simulink model "PowerWindowSystem"  (R2024b)
settings: Solver=VariableStepAuto  StartTime=0.0  StopTime=20  RelTol=1e-3  AbsTol=1e-3  EnableMultiTasking=on
libraries: fl_lib x26, sdl_lib x10, nesl_utility x5
CloseFcn:
  | try,close(h1_PowerWindowSystem),end
  | clear h1_PowerWindowSystem
  | 
  | 
  | clear simlog_PowerWindowSystem
Description:
  | Power Window System
settings Model: Creator=The MathWorks, Inc.  LastModifiedBy=linus
settings SolverCC: AutoScaleAbsTol=off  MaxConsecutiveMinStep=5  AlgebraicLoopSolver=TrustRegion  MaxZcPerStep=1
settings DataIOCC: LimitDataPoints=on  MaxDataPoints=10000  SaveFormat=Array  ReturnWorkspaceOutputs=off  SignalLoggingName=logsout_PowerWindowSystem
settings OptimizationCC: ExpressionDepthLimit=2147483647  EfficientMapNaN2IntZero=off  LifeSpan=inf
settings DebuggingCC: UnconnectedInputMsg=warning  UnconnectedOutputMsg=warning  UnconnectedLineMsg=warning  StateNameClashWarn=warning  PregeneratedLibrarySubsystemCodeDiagnostic=none  SFUnexpectedBacktrackingDiag=warning  SFNoUnconditionalDefaultTransitionDiag=warning  SFExecutionAtInitializationDiag=none  ArithmeticOperatorsInVariantConditions=warning
settings HardwareCC: ProdBitPerPointer=32  ProdBitPerSizeT=32  ProdBitPerPtrDiffT=32  ProdLargestAtomicFloat=None  ProdIntDivRoundTo=Undefined  ProdEndianess=Unspecified  ProdWordSize=32  ProdHWDeviceType=32-bit Generic
settings ModelReferenceCC: EnableRefExpFcnMdlSchedulingChecks=on  PropagateSignalLabelsOutOfModel=off
settings SFSimCC: SimUseLocalCustomCode=off  CustomCodeUndefinedFunction=UseInterfaceOnly
settings RTWCC: RTWUseLocalCustomCode=off  GPUComputeCapability=3.5  DLArmComputeVersion=19.05
settings CodeAppCC: StateflowObjectComments=on
settings GRTTargetCC: TargetLangStandard=C89/C90 (ANSI)  CombineOutputUpdateFcns=off  GRTInterface=on
settings ConfigComp: CovMetricSettings=dw  CovSaveCumulativeToWorkspaceVar=on  CovSaveSingleToWorkspaceVar=on  CovExternalEMLEnable=off
settings SimscapeCC: SimscapeLogType=all  SimscapeLogSimulationStatistics=on  SimscapeLogName=simlog_PowerWindowSystem  SimscapeLogDataHistory=20000

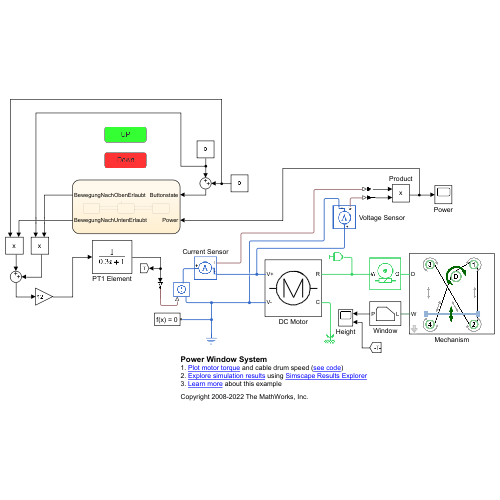
[thumbnail: Simulink's stored preview of the top-level diagram]
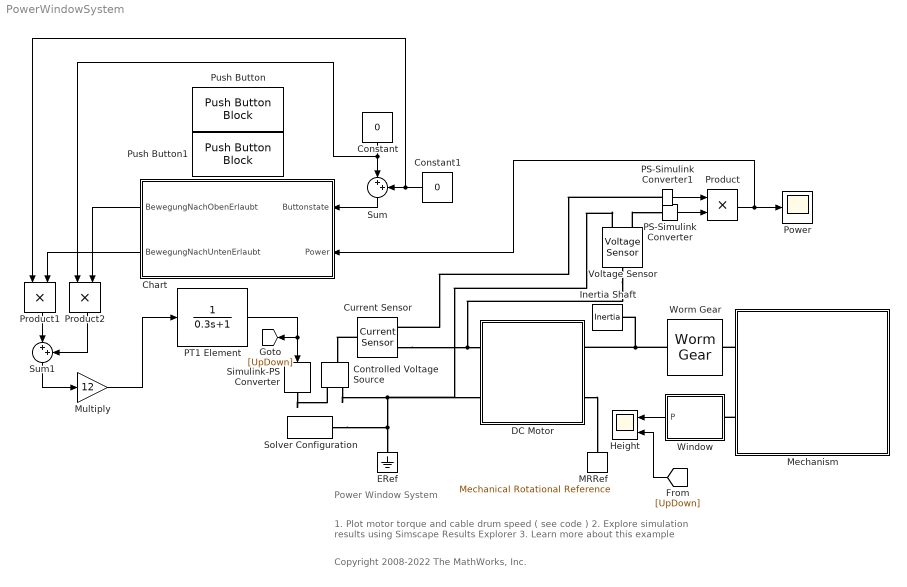
== system PowerWindowSystem ==
  note: Copyright 2008-2022 The MathWorks, Inc.
  note: Power Window System
  note: 1. Plot motor torque and cable drum speed ( see code )
      | 2. Explore simulation results using Simscape Results Explorer
      | 3. Learn more about this example
  Chart : Stateflow chart  TreatAsAtomicUnit=on
      settings: PortSchema="{\"entries\":[{\"content\":{\"sides\":[{\"content\":{\"connectorIds\":[\"In2\",\"In1\"]},\"type\":\"ConnectorPlacement.EquallySpacedRectSide\",\"uuid\":\"8bc5505b-9316-475f-ad7f-30c7afcbaf38\"},{\"content\":{\"connectorIds\":[\"Out1\",\"Out2\"],\"side\":\"RIGHT\"},\"type\":\"ConnectorPlacement.EquallySpacedRectSide\",\"uuid\":\"548d1c51-bdfb-47bd-abc9-5f518f35e423\"},{\"content\":{\"side\":\"TOP\"},\"type\":\"ConnectorPlacement.EquallySpacedRectSide\",\"uuid\":\"81f098c8-4566-4ae4-b1ae-e67fa706afd8\"}]},\"type\":\"ConnectorPlacement.EquallySpacedConnector\",\"uuid\":\"ae74842b-5900-4315-b481-75b4a04e7659\"}],\"packageUris\":[\"http://schema.mathworks.com/mf0/Connector/R2020b\"],\"version\":\"1.0\"}"
  Constant : Constant  Value=0
  Constant1 : Constant  Value=0
  Controlled Voltage Source : fl_lib/Electrical/Electrical Sources/Controlled Voltage Source
  Current Sensor : fl_lib/Electrical/Electrical Sensors/Current Sensor
  DC Motor : Subsystem  Tag=PublishSubsystem
      mask Display:
      | % Circle
      | plot(sin(0:0.1:2.2*pi)*0.9,cos(0:0.1:2.2*pi)*0.9);
      | 
      | % In/out
      | plot([-1.3 -0.9],[0 0]);
      | plot([1.3 0.9],[0 0]);
      | 
      | % 'M'
      | plot([0.5 0.5],[-0.5 0.5]);
      | plot([-0.5 -0.5],[-0.5 0.5]);
      | plot([0.5 0],[0.5 -0.5]);
      | plot([-0.5 0],[0.5 -0.5]);
      | 
      | % Plot points to set plot range
      | color('white');plot(1.5,1.5);plot(-1.5,-1.5)
      | color('black');
  ERef : fl_lib/Electrical/Electrical Elements/Electrical Reference
  Height : Scope  NumInputPorts=2
  Inertia Shaft : fl_lib/Mechanical/Rotational Elements/Inertia  inertia=0.01 kg*m^2  num_ports=foundation.enum.numPorts2.one  w_specify=on  w_priority=High  w=0 rad/s  w_nominal_specify=off  w_nominal_value=1  w_nominal_unit=rad/s  t_specify=off  t_priority=High  t=0 N*m  t_nominal_specify=off  t_nominal_value=1  t_nominal_unit=N*m
  MRRef : fl_lib/Mechanical/Rotational Elements/Mechanical Rotational Reference
  Mechanism : Subsystem  Tag=PublishSubsystem  mask(Power Window Cable Mechanism){pulley_rad=0.015, pulley_bearing_f=0.001, pulley_inertia=0.01, pulley_mus=0.5, pulley_vth=0.001, cable_massperlen=0.6, cable_k=5000, cable_b=500, cable_init_x=0.01, cable_guideway_f=10, drum_rad=0.030, drum_bearing_f=0.001*0.5}
      mask prompts: pulley_rad "Radius (m)"; pulley_bearing_f "Bearing Friction (N*m/(rad/s))"; pulley_inertia "Inertia (kg*m^2)"; pulley_mus "Static Friction with Belt"; pulley_vth "Friction Velocity Thresh. (m/s)"; cable_massperlen "Mass Per Length (kg/m)"; cable_k "Cable Stiffness (N/m)"; cable_b "Cable Damping (N/(m/s))"; cable_init_x "Cable Initial Deformation (m)"; cable_guideway_f "Guideway Friction (N/(m/s))"; drum_rad "Radius (m)"; drum_bearing_f "Bearing Friction (N*m/(rad/s))"
      mask help: Represents cable mechanism for raising and lowering a window. A cable is routed around four pulleys such that both ends of a lift plate can be raised and lowered. The mechanism is actuated by rotating the shaft of a rope drum.
      mask DialogControl Container28 Prompt: Pulley
      mask DialogControl Container25 Prompt: Cable
      mask DialogControl Container25_copy Prompt: Drum
      mask Display: image('PowerWindowSystemMechanismSchematic.jpg','center');
  Multiply : Gain  Gain=12
  PS-Simulink Converter : nesl_utility/PS-Simulink Converter  PhysicalDomain=network_engine_domain  SubClassName=ps_output  LeftPortType=input  RightPortType=output  PseudoPeriodic=off  Frequencies=[]  VectorFormat=inherit  Unit=inherit  AffineConversion=off
  PS-Simulink Converter1 : nesl_utility/PS-Simulink Converter  PhysicalDomain=network_engine_domain  SubClassName=ps_output  LeftPortType=input  RightPortType=output  PseudoPeriodic=off  Frequencies=[]  VectorFormat=inherit  Unit=inherit  AffineConversion=off
  PT1 Element : TransferFcn  Denominator=[0.3 1]
  Power : Scope
  Product : Product
  Product1 : Product
  Product2 : Product
  Push Button : PushButtonBlock  ButtonText=UP  OnValue=-1  OffValue=0.000000
  Push Button1 : PushButtonBlock  ButtonText=Down  OffValue=0.000000
  Simulink-PS Converter : nesl_utility/Simulink-PS Converter  PhysicalDomain=network_engine_domain  SubClassName=ps_input  LeftPortType=input  RightPortType=output  PseudoPeriodic=off  Frequencies=[]  NoiseDistribution=none  NoiseParameters=[]  Unit=V  AffineConversion=off  FilteringAndDerivatives=filter  SimscapeFilterOrder=1  InputFilterTimeConstant=0.1  UdotUserProvided=1
  Solver Configuration : nesl_utility/Solver Configuration  PhysicalDomain=network_engine_domain  SubClassName=solver  LeftPortType=input  RightPortType=generic  Tones=[]  Harmonics=[]  SimulateNoise=off  Profile=off  UseLocalSampling=off  EnableSwitchedLinearOptims=on  FrequencyDomain=off  UseCCode=off  RelTol=0.001  AbsTol=1e-06  MinStep=1e-09  ToWorkspace=off  RevertToSquareIcSolve=off  NumHomotopyIterations=100  PhasorMode=off  PhasorModeNumHarmonics=1  ConsistencySolver=NEWTON_XTOL_AFTER_FTOL  IndexReductionMethod=DerivativeReplacement  DoDC=off  ResidualTolerance=1e-9  ConsistencyTolSource=GLOBAL  ConsistencyAbsTol=0.001  ConsistencyRelTol=0.001  ConsistencyTolFactor=0.001  UseLocalSolver=off  LocalSolverChoice=NE_PARTITIONING_ADVANCER  ResolveIndetEquations=on  FunctionEvalNumThread=1  LocalSolverSampleTime=.001  DoFixedCost=off  MaxNonlinIter=6  MaxModeIter=2  ComputeImpulses=off  ImpulseIterations=2  LinearAlgebra=auto  LinearAlgebraNumThread=0  EquationFormulation=NE_TIME_EF  DelaysMemoryBudget=1024  AutomaticFiltering=on  FilteringTimeConstant=0.001  PartitionStorageMethod=EXHAUSTIVE  PartitionMemoryBudget=1024  PartitionMethod=ROBUST  MultibodyUseLocalSolver=off  MultibodyLocalSolverChoice=ODE1  MultibodyLocalSolverSampleTime=0.001
  Sum : Sum  Inputs=|++
  Sum1 : Sum  Inputs=|++
  Voltage Sensor : fl_lib/Electrical/Electrical Sensors/Voltage Sensor
  Window : Subsystem  Tag=PublishSubsystem
      mask Display:
      | patch([-1 -1 1 1 -1]*10,[-1 1 1 -1 -1]*8,[1 1 1]);
      | 
      | plot([1 -1]*6,[-1 -1]*5)
      | plot([1 1]*6,[-1 0.6]*5);
      | plot([1 0.8]*6,[0.6 0.9]*5);
      | plot([0.8 -0.1]*6,[0.9 0.9]*5);
      | plot([-0.1 -1]*6,[0.9 0]*5);
      | plot([-1 -1]*6,[0 -1]*5);
  Worm Gear : sdl_lib/Gears/Worm Gear  ratio=50  thread_type=1  friction_model=2  friction_parameterization=1  pr_ang=17.5 deg  lead_ang=3 deg  fr_coeff=0.2  eff_wg=0.74  eff_gw=0.65  temperature_TLU=[ 280 300 320 ] K  efficiency_wg_TLU=[ 0.75 0.7 0.65 ]  efficiency_gw_TLU=[ 0.5 0.45 0.4 ]  pwr_thr=0.001 W  mu_visc=[ 0.001 0.001 ] N*m/(rad/s)  thermal_mass=50 J/K  temperature_specify=off  temperature_priority=High  temperature=300 K  temperature_nominal_specify=off  temperature_nominal_value=1  temperature_nominal_unit=K
      settings: InternalSimscapePortConfiguration="{\"Bottom\":[],\"Left\":[{\"id\":\"W\",\"label\":\"W\",\"type\":\"foundation.mechanical.rotational.rotational\"}],\"Right\":[{\"id\":\"G\",\"label\":\"G\",\"type\":\"foundation.mechanical.rotational.rotational\"}],\"Top\":[]}"
  wires:
  Window/1(P) -> Height/1
  [UpDown] -> Height/2
  PS-Simulink Converter1/1 -> Product/1
  PS-Simulink Converter/1 -> Product/2
  Product/1 -> Chart/1(Power), Power/1
  Sum/1 -> Chart/2(Buttonstate)
  Sum1/1 -> Multiply/1
  Constant/1 -> Sum/1, Product2/1
  Constant1/1 -> Product1/1, Sum/2
  Chart/1(BewegungNachObenErlaubt) -> Product2/2
  Chart/2(BewegungNachUntenErlaubt) -> Product1/2
  Product1/1 -> Sum1/1
  Product2/1 -> Sum1/2
  Multiply/1 -> PT1 Element/1
  PT1 Element/1 -> Simulink-PS Converter/1, [UpDown]
  connections:
  Worm Gear/LConn1 -- DC Motor/RConn1 -- Inertia Shaft/LConn1
  Mechanism/LConn1 -- Worm Gear/RConn1
  Mechanism/LConn2 -- Window/LConn1
  DC Motor/RConn2 -- MRRef/LConn1
  Simulink-PS Converter/RConn1 -- Controlled Voltage Source/RConn1
  Controlled Voltage Source/RConn2 -- Voltage Sensor/RConn2 -- DC Motor/LConn2 -- ERef/LConn1 -- Solver Configuration/RConn1
  Voltage Sensor/RConn1 -- PS-Simulink Converter/LConn1
  PS-Simulink Converter1/LConn1 -- Current Sensor/RConn1
  Current Sensor/RConn2 -- Voltage Sensor/LConn1 -- DC Motor/LConn1
  Current Sensor/LConn1 -- Controlled Voltage Source/LConn1

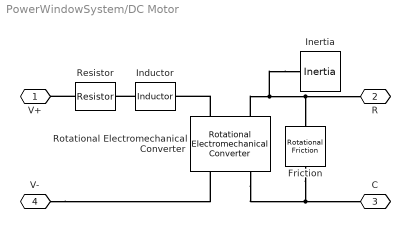
== system PowerWindowSystem/DC Motor ==
  Friction : fl_lib/Mechanical/Rotational Elements/Rotational Friction  brkwy_trq=0.02e-3 N*m  brkwy_vel=0.03347 rad/s  Col_trq=0.02e-3 N*m  visc_coef=.04 N*m/(rad/s)  w_specify=off  w_priority=High  w=0 rad/s  w_nominal_specify=off  w_nominal_value=1  w_nominal_unit=rad/s  t_specify=off  t_priority=High  t=0 N*m  t_nominal_specify=off  t_nominal_value=1  t_nominal_unit=N*m
  Inductor : fl_lib/Electrical/Electrical Elements/Inductor  l=5.5e-5 H  r=0 Ohm  g=1e-09 1/Ohm  i_specify=off  i_priority=High  i=0 A  i_nominal_specify=off  i_nominal_value=1  i_nominal_unit=A  v_specify=off  v_priority=High  v=0 V  v_nominal_specify=off  v_nominal_value=1  v_nominal_unit=V  i_L_specify=off  i_L_priority=High  i_L=0 A  i_L_nominal_specify=off  i_L_nominal_value=1  i_L_nominal_unit=A
  Inertia : fl_lib/Mechanical/Rotational Elements/Inertia  inertia=2.5e-5 g*cm^2  num_ports=foundation.enum.numPorts2.one  w_specify=on  w_priority=None  w=0 rad/s  w_nominal_specify=off  w_nominal_value=1  w_nominal_unit=rad/s  t_specify=off  t_priority=High  t=0 N*m  t_nominal_specify=off  t_nominal_value=1  t_nominal_unit=N*m
  Resistor : fl_lib/Electrical/Electrical Elements/Resistor  Tag=Factory Generic  R=.05 Ohm  i_specify=off  i_priority=High  i=0 A  i_nominal_specify=off  i_nominal_value=1  i_nominal_unit=A  v_specify=off  v_priority=High  v=0 V  v_nominal_specify=off  v_nominal_value=1  v_nominal_unit=V
  Rotational Electromechanical Converter : fl_lib/Electrical/Electrical Elements/Rotational Electromechanical Converter  K=.015 V/rpm  i_specify=off  i_priority=High  i=0 A  i_nominal_specify=off  i_nominal_value=1  i_nominal_unit=A  v_specify=off  v_priority=High  v=0 V  v_nominal_specify=off  v_nominal_value=1  v_nominal_unit=V  t_specify=off  t_priority=High  t=0 N*m  t_nominal_specify=off  t_nominal_value=1  t_nominal_unit=N*m  w_specify=off  w_priority=High  w=0 rad/s  w_nominal_specify=off  w_nominal_value=1  w_nominal_unit=rad/s
  V+ : PMIOPort  Side=Left
  R : PMIOPort  Port=2  Side=Right
  C : PMIOPort  Port=3  Side=Right
  V- : PMIOPort  Port=4  Side=Left
  connections:
  Rotational Electromechanical Converter/RConn2 -- C/RConn1 -- Friction/RConn1
  Inertia/LConn1 -- R/RConn1 -- Friction/LConn1 -- Rotational Electromechanical Converter/LConn2
  Inductor/LConn1 -- Resistor/RConn1
  Resistor/LConn1 -- V+/RConn1
  V-/RConn1 -- Rotational Electromechanical Converter/RConn1
  Rotational Electromechanical Converter/LConn1 -- Inductor/RConn1

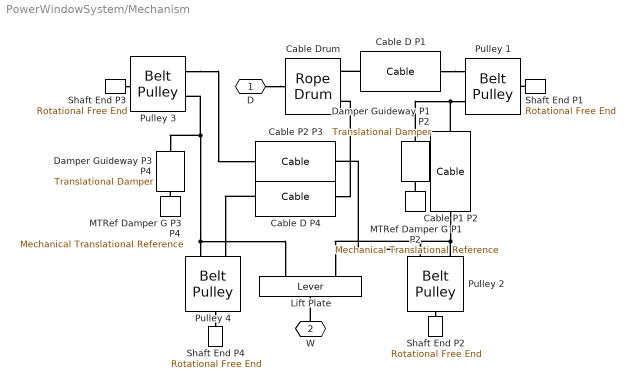
== system PowerWindowSystem/Mechanism ==
  Cable D P1 : sdl_lib/Couplings & Drives/Cable  model_variable_rest_length=false  minimum_rest_length=0.01 m  stretch_parameterization=sdl.enum.CableStretch.Constant  stiffness=cable_k N/m  rigidity=1000 N  damping=cable_b N/(m/s)  stretch_vector=[.1, .2, .5, 1] m  stiffness_vector=[500, 520, 540, 540] N/m  damping_vector=[50, 60, 80, 80] N*s/m  rest_length_vector=[.25, .5, 1] m  stretch_per_rest_length_vector=[.01, .02, .1, .25]  stiffness_table=[500, 600, 600, 500; 250, 300, 300, 250; 125, 150, 150, 125] N/m  damping_table=[50, 60, 60, 50; 50, 60, 60, 50; 50, 60, 60, 50] N*s/m  model_slack=false  slack_model=sdl.enum.SlackBoundary.smooth  transition=0.1 mm  model_mass=simscape.enum.onoff.off  mass=1 kg  linear_density=0.2 kg/m  model_gravity=false  gravity=9.81 m/s^2  theta=0 deg  check_tension=simscape.enum.onoff.on  breakable=sdl.enum.max_tension.off  f_max=1e5 N  s_specify=on  s_priority=High  s=cable_init_x m  s_nominal_specify=off  s_nominal_value=1  s_nominal_unit=m  v_specify=off  v_priority=None  v=0 m/s  v_nominal_specify=off  v_nominal_value=1  v_nominal_unit=m/s  f_specify=off  f_priority=None  f=0 N  f_nominal_specify=off  f_nominal_value=1  f_nominal_unit=N  f_mass_B_specify=off  f_mass_B_priority=None  f_mass_B=0 N  f_mass_B_nominal_specify=off  f_mass_B_nominal_value=1  f_mass_B_nominal_unit=N  f_mass_F_specify=off  f_mass_F_priority=None  f_mass_F=0 N  f_mass_F_nominal_specify=off  f_mass_F_nominal_value=1  f_mass_F_nominal_unit=N
      settings: InternalSimscapePortConfiguration="{\"Bottom\":[],\"Left\":[{\"id\":\"B\",\"label\":\"B\",\"type\":\"foundation.mechanical.translational.translational\"}],\"Right\":[{\"id\":\"F\",\"label\":\"F\",\"type\":\"foundation.mechanical.translational.translational\"}],\"Top\":[]}"
  Cable D P4 : sdl_lib/Couplings & Drives/Cable  model_variable_rest_length=false  minimum_rest_length=0.01 m  stretch_parameterization=sdl.enum.CableStretch.Constant  stiffness=cable_k N/m  rigidity=1000 N  damping=cable_b N/(m/s)  stretch_vector=[.1, .2, .5, 1] m  stiffness_vector=[500, 520, 540, 540] N/m  damping_vector=[50, 60, 80, 80] N*s/m  rest_length_vector=[.25, .5, 1] m  stretch_per_rest_length_vector=[.01, .02, .1, .25]  stiffness_table=[500, 600, 600, 500; 250, 300, 300, 250; 125, 150, 150, 125] N/m  damping_table=[50, 60, 60, 50; 50, 60, 60, 50; 50, 60, 60, 50] N*s/m  model_slack=false  slack_model=sdl.enum.SlackBoundary.smooth  transition=0.1 mm  model_mass=simscape.enum.onoff.off  mass=1 kg  linear_density=0.2 kg/m  model_gravity=false  gravity=9.81 m/s^2  theta=0 deg  check_tension=simscape.enum.onoff.on  breakable=sdl.enum.max_tension.off  f_max=1e5 N  s_specify=on  s_priority=High  s=cable_init_x m  s_nominal_specify=off  s_nominal_value=1  s_nominal_unit=m  v_specify=off  v_priority=None  v=0 m/s  v_nominal_specify=off  v_nominal_value=1  v_nominal_unit=m/s  f_specify=off  f_priority=None  f=0 N  f_nominal_specify=off  f_nominal_value=1  f_nominal_unit=N  f_mass_B_specify=off  f_mass_B_priority=None  f_mass_B=0 N  f_mass_B_nominal_specify=off  f_mass_B_nominal_value=1  f_mass_B_nominal_unit=N  f_mass_F_specify=off  f_mass_F_priority=None  f_mass_F=0 N  f_mass_F_nominal_specify=off  f_mass_F_nominal_value=1  f_mass_F_nominal_unit=N
      settings: InternalSimscapePortConfiguration="{\"Bottom\":[],\"Left\":[{\"id\":\"B\",\"label\":\"B\",\"type\":\"foundation.mechanical.translational.translational\"}],\"Right\":[{\"id\":\"F\",\"label\":\"F\",\"type\":\"foundation.mechanical.translational.translational\"}],\"Top\":[]}"
  Cable Drum : sdl_lib/Couplings & Drives/Rope Drum  r_drum=drum_rad m  windup=sdl.enum.belt_direction.same  check_tension=sdl.enum.tension_check.off  b_drum=drum_bearing_f N*m/(rad/s)  model_inertia=sdl.enum.model_inertia.off  inertia=0.01 kg*m^2  initial_velocity=0 rad/s
      settings: InternalSimscapePortConfiguration="{\"Bottom\":[],\"Left\":[{\"id\":\"S\",\"label\":\"S\",\"type\":\"foundation.mechanical.rotational.rotational\"}],\"Right\":[{\"id\":\"A\",\"label\":\"A\",\"type\":\"foundation.mechanical.translational.translational\"},{\"id\":\"B\",\"label\":\"B\",\"type\":\"foundation.mechanical.translational.translational\"}],\"Top\":[]}"
  Cable P1 P2 : sdl_lib/Couplings & Drives/Cable  model_variable_rest_length=false  minimum_rest_length=0.01 m  stretch_parameterization=sdl.enum.CableStretch.Constant  stiffness=cable_k N/m  rigidity=1000 N  damping=cable_b N/(m/s)  stretch_vector=[.1, .2, .5, 1] m  stiffness_vector=[500, 520, 540, 540] N/m  damping_vector=[50, 60, 80, 80] N*s/m  rest_length_vector=[.25, .5, 1] m  stretch_per_rest_length_vector=[.01, .02, .1, .25]  stiffness_table=[500, 600, 600, 500; 250, 300, 300, 250; 125, 150, 150, 125] N/m  damping_table=[50, 60, 60, 50; 50, 60, 60, 50; 50, 60, 60, 50] N*s/m  model_slack=false  slack_model=sdl.enum.SlackBoundary.smooth  transition=0.1 mm  model_mass=simscape.enum.onoff.off  mass=1 kg  linear_density=0.2 kg/m  model_gravity=false  gravity=9.81 m/s^2  theta=0 deg  check_tension=simscape.enum.onoff.on  breakable=sdl.enum.max_tension.off  f_max=1e5 N  s_specify=on  s_priority=High  s=cable_init_x m  s_nominal_specify=off  s_nominal_value=1  s_nominal_unit=m  v_specify=off  v_priority=None  v=0 m/s  v_nominal_specify=off  v_nominal_value=1  v_nominal_unit=m/s  f_specify=off  f_priority=None  f=0 N  f_nominal_specify=off  f_nominal_value=1  f_nominal_unit=N  f_mass_B_specify=off  f_mass_B_priority=None  f_mass_B=0 N  f_mass_B_nominal_specify=off  f_mass_B_nominal_value=1  f_mass_B_nominal_unit=N  f_mass_F_specify=off  f_mass_F_priority=None  f_mass_F=0 N  f_mass_F_nominal_specify=off  f_mass_F_nominal_value=1  f_mass_F_nominal_unit=N
      settings: InternalSimscapePortConfiguration="{\"Bottom\":[],\"Left\":[{\"id\":\"B\",\"label\":\"B\",\"type\":\"foundation.mechanical.translational.translational\"}],\"Right\":[{\"id\":\"F\",\"label\":\"F\",\"type\":\"foundation.mechanical.translational.translational\"}],\"Top\":[]}"
  Cable P2 P3 : sdl_lib/Couplings & Drives/Cable  model_variable_rest_length=false  minimum_rest_length=0.01 m  stretch_parameterization=sdl.enum.CableStretch.Constant  stiffness=cable_k N/m  rigidity=1000 N  damping=cable_b N/(m/s)  stretch_vector=[.1, .2, .5, 1] m  stiffness_vector=[500, 520, 540, 540] N/m  damping_vector=[50, 60, 80, 80] N*s/m  rest_length_vector=[.25, .5, 1] m  stretch_per_rest_length_vector=[.01, .02, .1, .25]  stiffness_table=[500, 600, 600, 500; 250, 300, 300, 250; 125, 150, 150, 125] N/m  damping_table=[50, 60, 60, 50; 50, 60, 60, 50; 50, 60, 60, 50] N*s/m  model_slack=false  slack_model=sdl.enum.SlackBoundary.smooth  transition=0.1 mm  model_mass=simscape.enum.onoff.off  mass=1 kg  linear_density=0.2 kg/m  model_gravity=false  gravity=9.81 m/s^2  theta=0 deg  check_tension=false  breakable=sdl.enum.max_tension.off  f_max=1e5 N  s_specify=on  s_priority=High  s=cable_init_x m  s_nominal_specify=off  s_nominal_value=1  s_nominal_unit=m  v_specify=off  v_priority=None  v=0 m/s  v_nominal_specify=off  v_nominal_value=1  v_nominal_unit=m/s  f_specify=off  f_priority=None  f=0 N  f_nominal_specify=off  f_nominal_value=1  f_nominal_unit=N  f_mass_B_specify=off  f_mass_B_priority=None  f_mass_B=0 N  f_mass_B_nominal_specify=off  f_mass_B_nominal_value=1  f_mass_B_nominal_unit=N  f_mass_F_specify=off  f_mass_F_priority=None  f_mass_F=0 N  f_mass_F_nominal_specify=off  f_mass_F_nominal_value=1  f_mass_F_nominal_unit=N
      settings: InternalSimscapePortConfiguration="{\"Bottom\":[],\"Left\":[{\"id\":\"B\",\"label\":\"B\",\"type\":\"foundation.mechanical.translational.translational\"}],\"Right\":[{\"id\":\"F\",\"label\":\"F\",\"type\":\"foundation.mechanical.translational.translational\"}],\"Top\":[]}"
  Damper Guideway P1 P2 : fl_lib/Mechanical/Translational Elements/Translational Damper  D=cable_guideway_f N/(m/s)  v_specify=off  v_priority=High  v=0 m/s  v_nominal_specify=off  v_nominal_value=1  v_nominal_unit=m/s  f_specify=off  f_priority=High  f=0 N  f_nominal_specify=off  f_nominal_value=1  f_nominal_unit=N
  Damper Guideway P3 P4 : fl_lib/Mechanical/Translational Elements/Translational Damper  D=cable_guideway_f N/(m/s)  v_specify=off  v_priority=High  v=0 m/s  v_nominal_specify=off  v_nominal_value=1  v_nominal_unit=m/s  f_specify=off  f_priority=High  f=0 N  f_nominal_specify=off  f_nominal_value=1  f_nominal_unit=N
  Lift Plate : fl_lib/Mechanical/Mechanisms/Lever  arm_AC=0.25 m  arm_BC=0.25 m  f_A_specify=off  f_A_priority=High  f_A=0 N  f_A_nominal_specify=off  f_A_nominal_value=1  f_A_nominal_unit=N  f_B_specify=off  f_B_priority=High  f_B=0 N  f_B_nominal_specify=off  f_B_nominal_value=1  f_B_nominal_unit=N  f_C_specify=off  f_C_priority=High  f_C=0 N  f_C_nominal_specify=off  f_C_nominal_value=1  f_C_nominal_unit=N
      settings: InternalSimscapePortConfiguration="{\"Bottom\":[],\"Left\":[{\"id\":\"A\",\"label\":\"A\",\"type\":\"foundation.mechanical.translational.translational\"},{\"id\":\"B\",\"label\":\"B\",\"type\":\"foundation.mechanical.translational.translational\"}],\"Right\":[{\"id\":\"C\",\"label\":\"C\",\"type\":\"foundation.mechanical.translational.translational\"}],\"Top\":[]}"
  MTRef Damper G P1 P2 : fl_lib/Mechanical/Translational Elements/Mechanical Translational Reference
  MTRef Damper G P3 P4 : fl_lib/Mechanical/Translational Elements/Mechanical Translational Reference
  Pulley 1 : sdl_lib/Couplings & Drives/Belt Pulley  belt_type=sdl.enum.belt_type.flat  sheave_ang=30 deg  num_belts=1  model_f_c=sdl.enum.model_centrifugal.on  linear_density=cable_massperlen kg/m  belt_direction=sdl.enum.belt_direction.opposite  breakable=sdl.enum.max_tension.off  F_max=1e+5 N  check_tension=sdl.enum.tension_check.off  pulley_moveable=simscape.enum.onoff.off  r_pulley=pulley_rad m  b_pulley=pulley_bearing_f N*m/(rad/s)  model_inertia=sdl.enum.model_inertia.on  pulley_mass=0.01 kg  initial_vel=0 m/s  pulley_inertia=pulley_inertia kg*m^2  initial_velocity=0 rad/s  friction_model=sdl.enum.PulleyModel.Modal  initial_state_locked=sdl.enum.initial_lock.unlocked  mu=pulley_mus  mu_static=pulley_mus  mu_kinetic=pulley_mus * 0.85  phi_wrap=120 deg  v_thr=pulley_vth m/s  f_thr=0.01 N
      settings: InternalSimscapePortConfiguration="{\"Bottom\":[],\"Left\":[{\"id\":\"S\",\"label\":\"S\",\"type\":\"foundation.mechanical.rotational.rotational\"}],\"Right\":[{\"id\":\"A\",\"label\":\"A\",\"type\":\"foundation.mechanical.translational.translational\"},{\"id\":\"B\",\"label\":\"B\",\"type\":\"foundation.mechanical.translational.translational\"}],\"Top\":[]}"
  Pulley 2 : sdl_lib/Couplings & Drives/Belt Pulley  belt_type=sdl.enum.belt_type.flat  sheave_ang=30 deg  num_belts=1  model_f_c=sdl.enum.model_centrifugal.on  linear_density=cable_massperlen kg/m  belt_direction=sdl.enum.belt_direction.opposite  breakable=sdl.enum.max_tension.off  F_max=1e+5 N  check_tension=sdl.enum.tension_check.off  pulley_moveable=simscape.enum.onoff.off  r_pulley=pulley_rad m  b_pulley=pulley_bearing_f N*m/(rad/s)  model_inertia=sdl.enum.model_inertia.on  pulley_mass=0.01 kg  initial_vel=0 m/s  pulley_inertia=pulley_inertia kg*m^2  initial_velocity=0 rad/s  friction_model=sdl.enum.PulleyModel.Modal  initial_state_locked=sdl.enum.initial_lock.unlocked  mu=pulley_mus  mu_static=pulley_mus  mu_kinetic=pulley_mus * 0.85  phi_wrap=145 deg  v_thr=pulley_vth m/s  f_thr=0.01 N
      settings: InternalSimscapePortConfiguration="{\"Bottom\":[],\"Left\":[{\"id\":\"S\",\"label\":\"S\",\"type\":\"foundation.mechanical.rotational.rotational\"}],\"Right\":[{\"id\":\"A\",\"label\":\"A\",\"type\":\"foundation.mechanical.translational.translational\"},{\"id\":\"B\",\"label\":\"B\",\"type\":\"foundation.mechanical.translational.translational\"}],\"Top\":[]}"
  Pulley 3 : sdl_lib/Couplings & Drives/Belt Pulley  belt_type=sdl.enum.belt_type.flat  sheave_ang=30 deg  num_belts=1  model_f_c=sdl.enum.model_centrifugal.on  linear_density=cable_massperlen kg/m  belt_direction=sdl.enum.belt_direction.opposite  breakable=sdl.enum.max_tension.off  F_max=1e+5 N  check_tension=sdl.enum.tension_check.off  pulley_moveable=simscape.enum.onoff.off  r_pulley=pulley_rad m  b_pulley=pulley_bearing_f N*m/(rad/s)  model_inertia=sdl.enum.model_inertia.on  pulley_mass=0.01 kg  initial_vel=0 m/s  pulley_inertia=pulley_inertia kg*m^2  initial_velocity=0 rad/s  friction_model=sdl.enum.PulleyModel.Modal  initial_state_locked=sdl.enum.initial_lock.unlocked  mu=pulley_mus  mu_static=pulley_mus  mu_kinetic=pulley_mus * 0.85  phi_wrap=145 deg  v_thr=pulley_vth m/s  f_thr=0.01 N
      settings: InternalSimscapePortConfiguration="{\"Bottom\":[],\"Left\":[{\"id\":\"S\",\"label\":\"S\",\"type\":\"foundation.mechanical.rotational.rotational\"}],\"Right\":[{\"id\":\"A\",\"label\":\"A\",\"type\":\"foundation.mechanical.translational.translational\"},{\"id\":\"B\",\"label\":\"B\",\"type\":\"foundation.mechanical.translational.translational\"}],\"Top\":[]}"
  Pulley 4 : sdl_lib/Couplings & Drives/Belt Pulley  belt_type=sdl.enum.belt_type.flat  sheave_ang=30 deg  num_belts=1  model_f_c=sdl.enum.model_centrifugal.on  linear_density=cable_massperlen kg/m  belt_direction=sdl.enum.belt_direction.opposite  breakable=sdl.enum.max_tension.off  F_max=1e+5 N  check_tension=sdl.enum.tension_check.off  pulley_moveable=simscape.enum.onoff.off  r_pulley=pulley_rad m  b_pulley=pulley_bearing_f N*m/(rad/s)  model_inertia=sdl.enum.model_inertia.on  pulley_mass=0.01 kg  initial_vel=0 m/s  pulley_inertia=pulley_inertia kg*m^2  initial_velocity=0 rad/s  friction_model=sdl.enum.PulleyModel.Modal  initial_state_locked=sdl.enum.initial_lock.unlocked  mu=pulley_mus  mu_static=pulley_mus  mu_kinetic=pulley_mus * 0.85  phi_wrap=155 deg  v_thr=pulley_vth m/s  f_thr=0.01 N
      settings: InternalSimscapePortConfiguration="{\"Bottom\":[],\"Left\":[{\"id\":\"S\",\"label\":\"S\",\"type\":\"foundation.mechanical.rotational.rotational\"}],\"Right\":[{\"id\":\"A\",\"label\":\"A\",\"type\":\"foundation.mechanical.translational.translational\"},{\"id\":\"B\",\"label\":\"B\",\"type\":\"foundation.mechanical.translational.translational\"}],\"Top\":[]}"
  Shaft End P{1..4} (4 alike) : fl_lib/Mechanical/Rotational Elements/Rotational Free End  w_specify=off  w_priority=None  w=0 rad/s  w_nominal_specify=off  w_nominal_value=1  w_nominal_unit=rad/s
  D : PMIOPort  Side=Left
  W : PMIOPort  Port=2  Side=Left
  connections:
  W/RConn1 -- Lift Plate/RConn1
  D/RConn1 -- Cable Drum/LConn1
  MTRef Damper G P3 P4/LConn1 -- Damper Guideway P3 P4/RConn1
  Pulley 3/RConn1 -- Damper Guideway P3 P4/LConn1 -- Pulley 4/RConn1 -- Lift Plate/LConn1
  Shaft End P1/LConn1 -- Pulley 1/LConn1
  Pulley 2/LConn1 -- Shaft End P2/LConn1
  Shaft End P3/LConn1 -- Pulley 3/LConn1
  Pulley 4/LConn1 -- Shaft End P4/LConn1
  Pulley 2/RConn2 -- Cable P2 P3/RConn1
  Damper Guideway P1 P2/LConn1 -- Cable P1 P2/LConn1 -- Pulley 1/RConn1
  Pulley 2/RConn1 -- Cable P1 P2/RConn1 -- Lift Plate/LConn2
  MTRef Damper G P1 P2/LConn1 -- Damper Guideway P1 P2/RConn1
  Cable D P1/LConn1 -- Pulley 1/RConn2
  Cable D P1/RConn1 -- Cable Drum/RConn1
  Pulley 3/RConn2 -- Cable P2 P3/LConn1
  Cable D P4/RConn1 -- Pulley 4/RConn2
  Cable D P4/LConn1 -- Cable Drum/RConn2

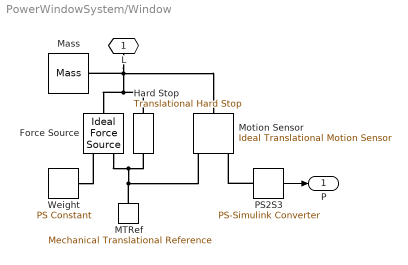
== system PowerWindowSystem/Window ==
  Force Source : fl_lib/Mechanical/Mechanical Sources/Ideal Force Source
  Hard Stop : fl_lib/Mechanical/Translational Elements/Translational Hard Stop  upper_bnd=0.3 m  lower_bnd=-0.1 m  model=3  stiff_up=1e+06 N/m  stiff_low=1e+06 N/m  D_up=150 N/(m/s)  D_low=150 N/(m/s)  transition=0.1 mm  coeff_rest=0.7  v_tol=0.001 m/s  f_tol=0.001 N  v_specify=off  v_priority=High  v=0 m/s  v_nominal_specify=off  v_nominal_value=1  v_nominal_unit=m/s  f_specify=off  f_priority=High  f=0 N  f_nominal_specify=off  f_nominal_value=1  f_nominal_unit=N  x_specify=on  x_priority=High  x=0 m  x_nominal_specify=off  x_nominal_value=1  x_nominal_unit=m  M_specify=off  M_priority=None  M=0
  MTRef : fl_lib/Mechanical/Translational Elements/Mechanical Translational Reference
  Mass : fl_lib/Mechanical/Translational Elements/Mass  mass=1.5 kg  num_ports=foundation.enum.numPorts2.one  v_specify=on  v_priority=High  v=0 m/s  v_nominal_specify=off  v_nominal_value=1  v_nominal_unit=m/s  f_specify=off  f_priority=High  f=0 N  f_nominal_specify=off  f_nominal_value=1  f_nominal_unit=N
  Motion Sensor : fl_lib/Mechanical/Mechanical Sensors/Ideal Translational Motion Sensor  reference=foundation.enum.MeasurementReference.difference  acceleration_port=false  velocity_port=true  position_port=true  offset=0 m
  PS2S3 : nesl_utility/PS-Simulink Converter  PhysicalDomain=network_engine_domain  SubClassName=ps_output  LeftPortType=input  RightPortType=output  PseudoPeriodic=off  Frequencies=[]  VectorFormat=1-D array  Unit=cm  AffineConversion=off
  Weight : fl_lib/Physical Signals/Sources/PS Constant  constant=-1.5 * 9.81
  L : PMIOPort  Side=Left
  P : Outport  VectorParamsAs1DForOutWhenUnconnected=off
  wires:
  PS2S3/1 -> P/1
  connections:
  MTRef/LConn1 -- Force Source/RConn2 -- Hard Stop/RConn1 -- Motion Sensor/RConn1
  Hard Stop/LConn1 -- L/RConn1 -- Motion Sensor/LConn1 -- Mass/LConn1 -- Force Source/LConn1
  Weight/RConn1 -- Force Source/RConn1
  PS2S3/LConn1 -- Motion Sensor/RConn3

== stateflow chart PowerWindowSystem/Chart ==
  state Geschlossen
    entry:
    BewegungNachUntenErlaubt = 1;
    BewegungNachObenErlaubt = 0;
  state Mittelposition
    entry:
    BewegungNachUntenErlaubt = 1;
    BewegungNachObenErlaubt = 1;
  state Offen
    entry:
    BewegungNachUntenErlaubt = 0;
    BewegungNachObenErlaubt = 1;
  (default) -> Mittelposition
  Mittelposition -> Geschlossen [order 1] : [Power > 266 && Buttonstate == -1]
  Mittelposition -> Offen [order 2] : [Power > 266 && Buttonstate == 1]
  Geschlossen -> Mittelposition : [Buttonstate == 1]
  Offen -> Mittelposition : [Buttonstate == -1]
  data: Power input; Buttonstate input; BewegungNachObenErlaubt output =1; BewegungNachUntenErlaubt output =1
